simulink model "MPC_gamecontroller_LiDAR"  (Simulink 7.6)
settings: Solver=ode3  StartTime=0.0  StopTime=inf  FixedStep=.05  RelTol=1e-3
InitFcn:
  | a2g = 1/9.81;
  | r2d = 180/pi;
  | K_sr = 15.97;
  | neutral_steer = 103;
  | s2t = (pi/180)*(1/K_sr);
  | A_kt =[         0         0         0         0         0         0
  |          0   -3.5058   -1.6990  -25.6114   -2.2435         0
  |          0    2.2782   -4.2575  -64.1772   -5.6218         0
  |          0         0    1.0000         0         0         0
  |          0   -0.0158    0.0295    0.4442   -4.1900         0
  |          0         0         0         0    1.0000         0];
  | 
  | 
  | B_kt =[0
  |    23.7845
  |   -16.0342
  |          0
  |    17.5770
  |          0];
  | 
  | dt = 0.05;
  | measnoise_posX = 3.36;
  | measnoise_posY = 3.95;
  | measnoise_theta = 0.136;
  | measnoise_phi =  0.078;
  | measnoise_velocity = measnoise_posX*dt;
  | 
  | accelnoiseX = 0.97;
  | accelnoiseY = 1.36;
  | gyronoisetheta = 0.04;
  | gyronoisephi = 0.021;
  | 
  | anx = accelnoiseX^2;
  | any = accelnoiseY^2;
  | anxy = accelnoiseX*accelnoiseY;
  | gntheta = gyronoisetheta^2;
  | agthetax = gyronoisetheta*accelnoiseX;
  | agthetay = gyronoisetheta*accelnoiseY;
  | gnphi = gyronoisephi^2;
  | agphix = gyronoisephi*accelnoiseX;
  | agphiy = gyronoisephi*accelnoiseY;
  | gnthetaphi = gyronoisetheta*gyronoisephi;
  | 
  | A = [1 dt 0 0 0 0;...
  |         0 1 0 0 0 0;...
  |         0 0 1 dt 0 0;...
  |         0 0 0 1 0 0;...
  |         0 0 0 0 1 0;...
  |         0 0 0 0 0 1];
  | 
  | Sw = [anx*dt^4/4, anx*dt^3/2, anxy*dt^4/4, anxy*dt^3/2,  agthetax*dt^3/2, agphix*dt^3/2;...
  |       anx*dt^3/2, anx*dt^2,   anxy*dt^3/2, anxy*dt^2, agthetax*dt^2,   agphix*dt^2;...
  |       anxy*dt^4/4, anxy*dt^3/2, any*dt^4/4, any*dt^3/2,  agthetay*dt^3/2, agphiy*dt^3/2;...
  |       anxy*dt^3/2, anxy*dt^2,   any*dt^3/2, any*dt^2, agthetay*dt^2, agphiy*dt^2;...
  |       agthetax*dt^3/2, agthetax*dt^2, agthetay*dt^3/2, agthetay*dt^2, gntheta*dt^2, gnthetaphi*dt^2;...
  |       agphix*dt^3/2, agphix*dt^2, agphiy*dt^3/2, agphiy*dt^2, gnthetaphi*dt^2, gnphi*dt^2];
  | 
  | Sz =  [measnoise_posX^2, 0, 0, 0, 0, 0;...
  |          0, measnoise_velocity^2, 0, 0, 0, 0;...
  |          0, 0, measnoise_posY^2, 0, 0, 0;...
  |          0, 0, 0, measnoise_velocity^2, 0, 0;...
  |          0, 0, 0, 0, measnoise_theta^2, 0;...
  |          0, 0, 0, 0, 0, measnoise_phi^2];
  | 
  | load MPC_test_2
StartFcn:
  | Threshold = 12;
  | MaxCluster = 75;
  | Num_Beams = 726;
  | Road_Width = 10.25;
  | Cone_Area = 0.125;
  | Cone_Spacing = 4.42;
  | Scaling = 1.1;
  | areaBuffer = 0.125;
  | spacingBuffer = 0.035;
  | RoadfromConeoffset = 0.3;
  | threatThreshold = 1;
  | distThreshold = 10;
  | minSpeed = 2.0;
  | minDistance = 1.0;
  | threatConeAngle = 75;
  | allowableDistToCone = .01;
  | thresholdManueverAngle = 80;
  | maxStepSize = 1.0;
  | aspectRatioBuffer = 1;
  | javaaddpath({'/'});
  | import ClusterMethodWithFinal.*;
  | %import ClusterMethodWithNoFlicker.*;
  | %DataCluster = ClusterMethodWithNoFlicker(Threshold,MaxCluster,Scaling,...
  | %Road_Width,Cone_Area,Cone_Spacing,areaBuffer,spacingBuffer,RoadfromConeoffset,threatThreshold,...
  | %distThreshold,minSpeed,minDistance,threatConeAngle,allowableDistToCone,maxStepSize);
  | DataCluster = ClusterMethodWithFinal(Threshold,MaxCluster,Scaling,...
  | Road_Width,Cone_Area,Cone_Spacing,areaBuffer,spacingBuffer,RoadfromConeoffset,...
  | threatThreshold,distThreshold,minSpeed,minDistance,threatConeAngle,allowableDistToCone,...
  | thresholdManueverAngle,maxStepSize);
  | eml.extrinsic('evalin');
  | 
  | gd_scan(0);
StopFcn:
  | clear DataCluster;
  | clear Threshold;
  | clear MaxCluster;
  | clear Num_Beams;
  | clear Road_Width;
  | clear Cone_Area;
  | clear Cone_Spacing;
  | clear Scaling;
  | clear areaBuffer;
  | clear spacingBuffer;
  | clear RoadfromConeoffset;
  | clear threatThreshold;
  | clear distThreshold;
  | clear minSpeed;
  | clear minDistance;
  | clear threatConeAngle;
  | clear allowableDistToCone;
  | clear thresholdManueverAngle;
  | clear maxStepSize;
  | clear aspectRatioBuffer;
  | 
  | gd_scan(2);
undefined symbols (not defined in the file or in its folder): CR, serial
libraries: instrumentlib x3, realtime_pacer_lib x1, vrlib x1
settings Model: Creator=TCA  LastModifiedBy=ipainter  BufferReuse=off
settings OptimizationCC: BlockReduction=off  InlineParams=on  BufferReuse=off  InitFltsAndDblsToZero=on
settings DebuggingCC: AlgebraicLoopMsg=none  SolverPrmCheckMsg=none  InheritedTsInSrcMsg=none  UnconnectedInputMsg=none  UnconnectedOutputMsg=none  UnconnectedLineMsg=none  StrictBusMsg=Warning
settings SFSimCC: SimParseCustomCode=off

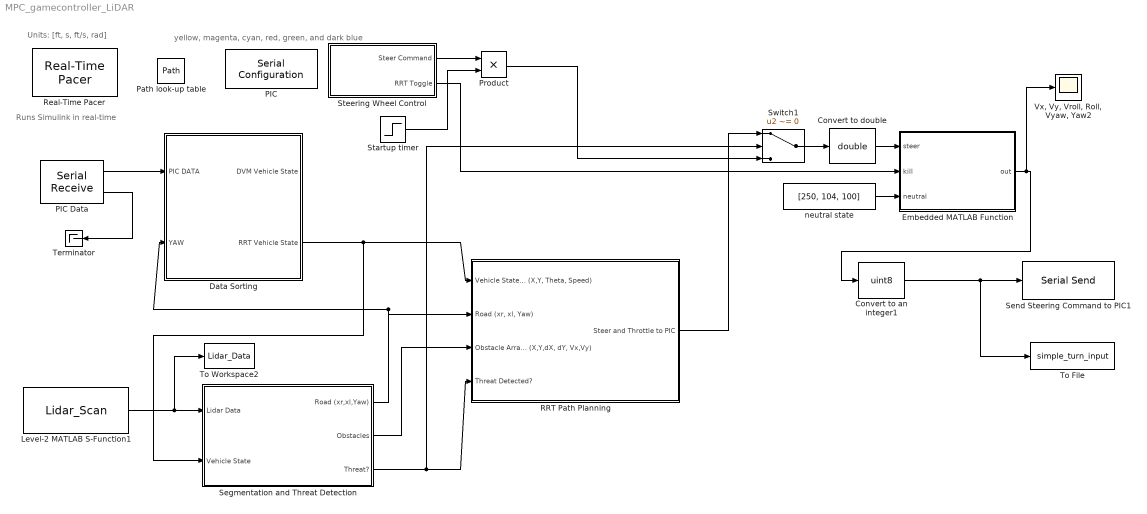
== system MPC_gamecontroller_LiDAR ==
  note: Runs Simulink
      |  in real-time
  note: Units: [ft, s, ft/s, rad]
  note: yellow, magenta, cyan, red, green, and dark blue
  Convert to an integer1 : DataTypeConversion  OutDataTypeStr=uint8  SampleTime=.05  SaturateOnIntegerOverflow=on  RndMeth=Zero
  Convert to double : DataTypeConversion  OutDataTypeStr=double  SampleTime=0.05  SaturateOnIntegerOverflow=on  RndMeth=Zero
  Data Sorting : Subsystem
  Embedded MATLAB Function : Stateflow chart  TreatAsAtomicUnit=on
  Level-2 MATLAB S-Function1 : M-S-Function  FunctionName=Lidar_Scan
  PIC : instrumentlib/Serial Configuration  Priority=-200000  DialogController=instrumentcreatedialog  DialogControllerArgs=DataTag0  ComPortMenu=<Please select a port...>  ComPort=COM5  ObjConstructor=serial('COM5');  BaudRate=9600  DataBits=8  Parity=none  StopBits=1  FlowControl=none  Timeout=10  ByteOrder=LittleEndian
  PIC Data : instrumentlib/Serial Receive  DialogController=instrumentcreatedialog  DialogControllerArgs=DataTag1  ComPortMenu=<Please select a port...>  ComPort=COM5  ObjConstructor=serial('COM5');  Terminator=CR ('\r')  DataSize="[1  16]"  DataType=uint8  EnableBlockingMode=off  ActionDataUnavailable=Output last received value  CustomValue=0  SampleTime=.05
  Path look-up table : DataStoreMemory  DataStoreName=Path  ReadBeforeWriteMsg=warning  WriteAfterWriteMsg=warning  WriteAfterReadMsg=warning  InitialValue=zeros(50, 6)  VectorParams1D=off
  Product : Product  RndMeth=Zero
  RRT Path Planning : Subsystem
  Real-Time Pacer : realtime_pacer_lib/Real-Time Pacer  simTimePerRealTime=1
  Segmentation and Threat Detection : Subsystem
  Send Steering Command to PIC1 : instrumentlib/Serial Send  DialogController=instrumentcreatedialog  DialogControllerArgs=DataTag2  ComPortMenu=<Please select a port...>  ComPort=COM5  ObjConstructor=serial('COM5');  Header=250  Terminator=<none>  EnableBlockingMode=off
  Startup timer : Step  Time=3  SampleTime=0
  Steering Wheel Control : Subsystem
  Switch1 : Switch  Criteria=u2 ~= 0
  Terminator : Terminator
  To File : ToFile  Filename=simple_turn_input  MatrixName=ST_input  SaveFormat=Timeseries
  To Workspace2 : ToWorkspace  VariableName=Lidar_Data  SampleTime=-1  SaveFormat=Structure With Time
  "Vx, Vy, Vroll, Roll, Vyaw, Yaw2" : Scope
      settings: TimeRange=10  YMax=30
  neutral state : Constant  Value=[250, 104, 100]
  wires:
  Convert to an integer1/1 -> To File/1, Send Steering Command to PIC1/1
  PIC Data/2 -> Terminator/1
  PIC Data/1 -> Data Sorting/1(PIC DATA)
  Segmentation and Threat Detection/2(Obstacles) -> RRT Path Planning/3("Obstacle Array (X,Y,dX, dY, Vx,Vy)")
  Segmentation and Threat Detection/1(Road (xr,xl,Yaw)) -> Data Sorting/2(" YAW"), RRT Path Planning/2("Road (xr, xl, Yaw)")
  RRT Path Planning/1(Steer and Throttle to PIC) -> Switch1/1
  Data Sorting/2(RRT Vehicle State) -> RRT Path Planning/1("Vehicle State (X,Y, Theta, Speed)"), Segmentation and Threat Detection/2(Vehicle State)
  neutral state/1 -> Embedded MATLAB Function/3(neutral)
  Embedded MATLAB Function/1(out) -> Convert to an integer1/1, "Vx, Vy, Vroll, Roll, Vyaw, Yaw2"/1
  Switch1/1 -> Convert to double/1
  Segmentation and Threat Detection/3(Threat?) -> Switch1/2, RRT Path Planning/4(Threat Detected?)
  Steering Wheel Control/1(Steer Command) -> Product/1
  Product/1 -> Switch1/3
  Startup timer/1 -> Product/2
  Steering Wheel Control/2(RRT Toggle) -> Embedded MATLAB Function/2(kill)
  Convert to double/1 -> Embedded MATLAB Function/1(steer)
  Level-2 MATLAB S-Function1/1 -> Segmentation and Threat Detection/1(Lidar Data), To Workspace2/1

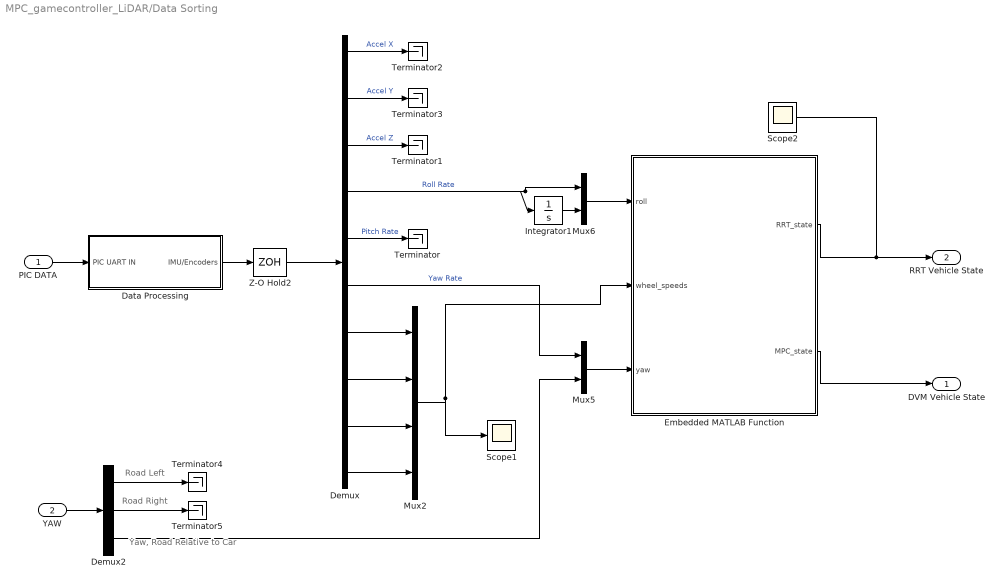
== system MPC_gamecontroller_LiDAR/Data Sorting ==
  note: Road Left
  note: Road Right
  note: Yaw, Road Relative to Car
  PIC DATA : Inport
  " YAW" : Inport  Port=2
  Data Processing : Subsystem
  Demux : Demux  Outputs=10
  Demux2 : Demux  Outputs=3
  Embedded MATLAB Function : Stateflow chart  TreatAsAtomicUnit=on
  Integrator1 : Integrator
  Mux2 : Mux
  Mux5 : Mux  Inputs=2
  Mux6 : Mux  Inputs=2
  Scope1 : Scope
      settings: SaveName=ScopeData3
  Scope2 : Scope
      settings: SaveName=ScopeData4
  Terminator{,1..5} (6 alike) : Terminator
  Z-O Hold2 : ZeroOrderHold  SampleTime=0.05
  DVM Vehicle State : Outport
  RRT Vehicle State : Outport  Port=2
  wires:
  Demux/6 -> Mux5/1  "Yaw Rate"
  Demux/2 -> Terminator3/1  "Accel Y"
  Demux/4 -> Mux6/1, Integrator1/1  "Roll Rate"
  Demux/5 -> Terminator/1  "Pitch Rate"
  Demux/7 -> Mux2/1
  Demux/8 -> Mux2/2
  Demux/9 -> Mux2/3
  Demux/10 -> Mux2/4
  Z-O Hold2/1 -> Demux/1
  Integrator1/1 -> Mux6/2
  Mux6/1 -> Embedded MATLAB Function/1(roll)
  Demux/1 -> Terminator2/1  "Accel X"
  Embedded MATLAB Function/2(MPC_state) -> DVM Vehicle State/1
  " YAW"/1 -> Demux2/1
  Demux/3 -> Terminator1/1  "Accel Z"
  Demux2/1 -> Terminator4/1
  Demux2/2 -> Terminator5/1
  Demux2/3 -> Mux5/2
  Mux5/1 -> Embedded MATLAB Function/3(yaw)
  Embedded MATLAB Function/1(RRT_state) -> RRT Vehicle State/1, Scope2/1
  Data Processing/1(IMU/Encoders) -> Z-O Hold2/1
  PIC DATA/1 -> Data Processing/1(PIC UART IN)
  Mux2/1 -> Embedded MATLAB Function/2(wheel_speeds), Scope1/1

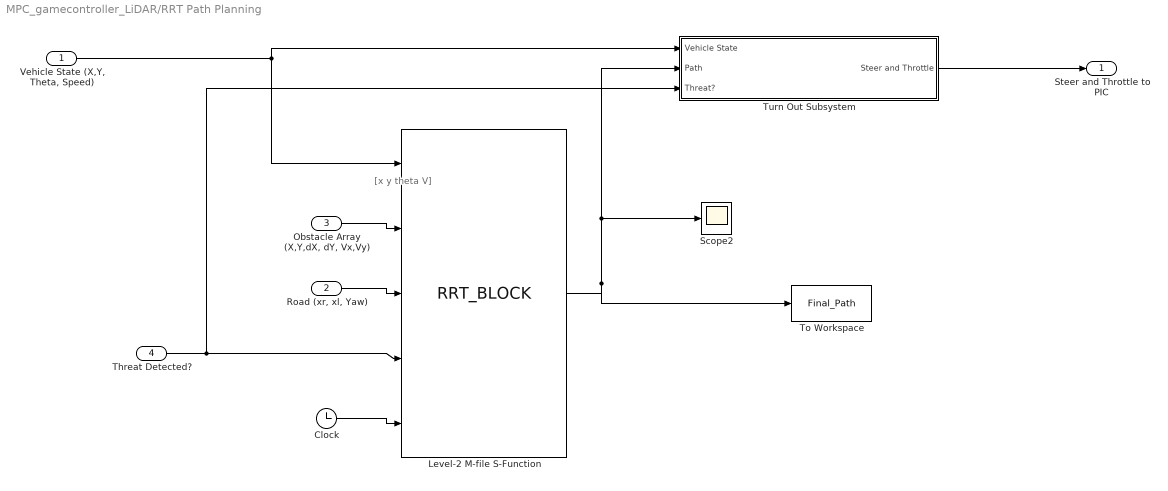
== system MPC_gamecontroller_LiDAR/RRT Path Planning ==
  note: [x y theta V]
  "Vehicle State (X,Y, Theta, Speed)" : Inport
  "Road (xr, xl, Yaw)" : Inport  Port=2
  "Obstacle Array (X,Y,dX, dY, Vx,Vy)" : Inport  Port=3
  Threat Detected? : Inport  Port=4
  Clock : Clock
      settings: Decimation=10
  Level-2 M-file S-Function : M-S-Function  FunctionName=RRT_BLOCK  Parameters=6
  Scope2 : Scope
      settings: SaveName=ScopeData5
  To Workspace : ToWorkspace  VariableName=Final_Path  SampleTime=-1  SaveFormat=Structure With Time
  Turn Out Subsystem : Subsystem
  Steer and Throttle to PIC : Outport
  wires:
  Clock/1 -> Level-2 M-file S-Function/5
  "Vehicle State (X,Y, Theta, Speed)"/1 -> Level-2 M-file S-Function/1, Turn Out Subsystem/1(Vehicle State)
  "Obstacle Array (X,Y,dX, dY, Vx,Vy)"/1 -> Level-2 M-file S-Function/2
  Turn Out Subsystem/1(Steer and Throttle) -> Steer and Throttle to PIC/1
  Threat Detected?/1 -> Level-2 M-file S-Function/4, Turn Out Subsystem/3(Threat?)
  "Road (xr, xl, Yaw)"/1 -> Level-2 M-file S-Function/3
  Level-2 M-file S-Function/1 -> Turn Out Subsystem/2(Path), Scope2/1, To Workspace/1

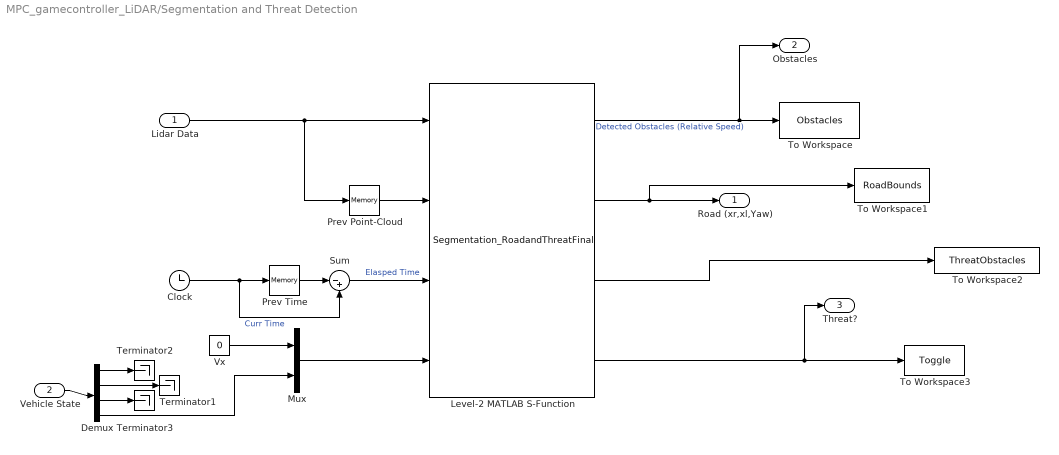
== system MPC_gamecontroller_LiDAR/Segmentation and Threat Detection ==
  Lidar Data : Inport
  Vehicle State : Inport  Port=2
  Clock : Clock
      settings: Decimation=10
  Demux : Demux
  Level-2 MATLAB S-Function : M-S-Function  FunctionName=Segmentation_RoadandThreatFinal
  Mux : Mux  Inputs=2
  Prev Point-Cloud : Memory
  Prev Time : Memory
  Sum : Sum  Inputs=|-+
  Terminator1 : Terminator
  Terminator2 : Terminator
  Terminator3 : Terminator
  To Workspace : ToWorkspace  VariableName=Obstacles  SampleTime=-1  SaveFormat=Structure With Time
  To Workspace1 : ToWorkspace  VariableName=RoadBounds  SampleTime=-1  SaveFormat=Structure With Time
  To Workspace2 : ToWorkspace  VariableName=ThreatObstacles  SampleTime=-1  SaveFormat=Structure With Time
  To Workspace3 : ToWorkspace  VariableName=Toggle  SampleTime=-1  SaveFormat=Structure With Time
  Vx : Constant  Value=0
  Road (xr,xl,Yaw) : Outport
  Obstacles : Outport  Port=2
  Threat? : Outport  Port=3
  wires:
  Prev Time/1 -> Sum/1
  Sum/1 -> Level-2 MATLAB S-Function/3  "Elasped Time"
  Clock/1 -> Prev Time/1, Sum/2  "Curr Time"
  Prev Point-Cloud/1 -> Level-2 MATLAB S-Function/2
  Level-2 MATLAB S-Function/1 -> To Workspace/1, Obstacles/1  "Detected Obstacles (Relative Speed)"
  Lidar Data/1 -> Prev Point-Cloud/1, Level-2 MATLAB S-Function/1
  Mux/1 -> Level-2 MATLAB S-Function/4
  Level-2 MATLAB S-Function/4 -> To Workspace3/1, Threat?/1
  Vx/1 -> Mux/1
  Vehicle State/1 -> Demux/1
  Demux/4 -> Mux/2
  Demux/1 -> Terminator2/1
  Demux/2 -> Terminator1/1
  Demux/3 -> Terminator3/1
  Level-2 MATLAB S-Function/2 -> Road (xr,xl,Yaw)/1, To Workspace1/1
  Level-2 MATLAB S-Function/3 -> To Workspace2/1

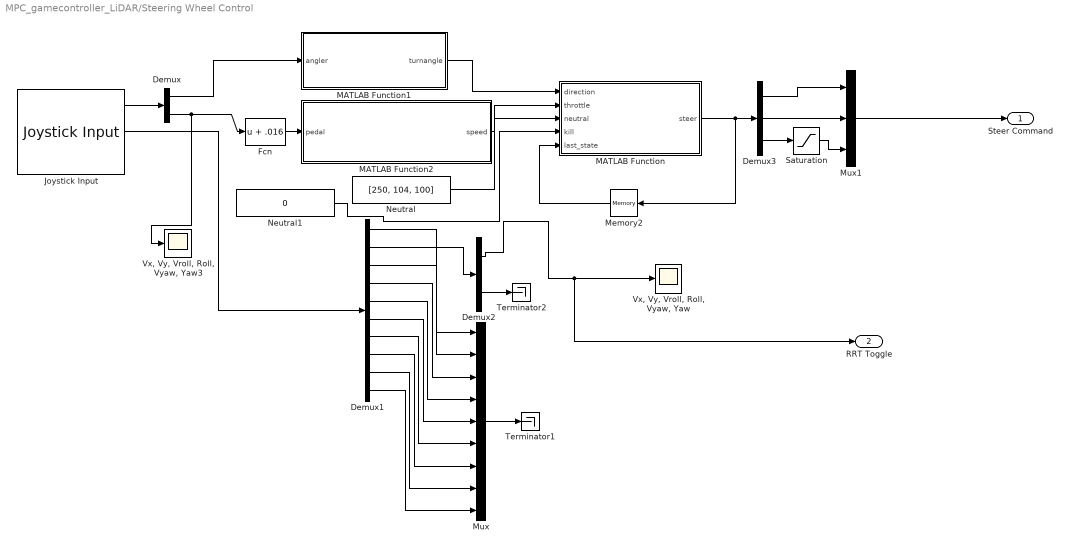
== system MPC_gamecontroller_LiDAR/Steering Wheel Control ==
  Demux : Demux  Outputs=2
  Demux1 : Demux  Outputs=10
  Demux2 : Demux  Outputs=2
  Demux3 : Demux  Outputs=3
  Fcn : Fcn  Expr=u + .016
  Joystick Input : vrlib/Joystick Input  joyid=1  adjustports=on  forcefeed=off
  MATLAB Function : Stateflow chart  TreatAsAtomicUnit=on
  MATLAB Function1 : Stateflow chart  TreatAsAtomicUnit=on
  MATLAB Function2 : Stateflow chart  TreatAsAtomicUnit=on
  Memory2 : Memory  X0=[250,104,100]  InheritSampleTime=on
  Mux : Mux  Inputs=9
  Mux1 : Mux  Inputs=3
  Neutral : Constant  Value=[250, 104, 100]
  Neutral1 : Constant  Value=0
  Saturation : Saturate  UpperLimit=200  LowerLimit=100
  Terminator1 : Terminator
  Terminator2 : Terminator
  "Vx, Vy, Vroll, Roll, Vyaw, Yaw" : Scope
      settings: TimeRange=10  YMax=30  SaveName=ScopeData7
  "Vx, Vy, Vroll, Roll, Vyaw, Yaw3" : Scope
      settings: TimeRange=10  YMax=30  SaveName=ScopeData6
  Steer Command : Outport
  RRT Toggle : Outport  Port=2
  wires:
  Joystick Input/1 -> Demux/1
  MATLAB Function2/1(speed) -> MATLAB Function/2(throttle)
  Neutral/1 -> MATLAB Function/3(neutral)
  Demux1/2 -> Demux2/1
  Demux2/1 -> "Vx, Vy, Vroll, Roll, Vyaw, Yaw"/1, RRT Toggle/1
  Demux2/2 -> Terminator2/1
  Demux1/1 -> Mux/1
  Demux1/3 -> Mux/2
  Demux1/4 -> Mux/3
  Demux1/5 -> Mux/4
  Demux1/6 -> Mux/5
  Demux1/7 -> Mux/6
  Demux1/8 -> Mux/7
  Demux1/9 -> Mux/8
  Demux1/10 -> Mux/9
  Mux/1 -> Terminator1/1
  Demux/2 -> "Vx, Vy, Vroll, Roll, Vyaw, Yaw3"/1, Fcn/1
  MATLAB Function1/1(turnangle) -> MATLAB Function/1(direction)
  Demux/1 -> MATLAB Function1/1(angler)
  Joystick Input/2 -> Demux1/1
  MATLAB Function/1(steer) -> Memory2/1, Demux3/1
  Memory2/1 -> MATLAB Function/5(last_state)
  Demux3/3 -> Saturation/1
  Saturation/1 -> Mux1/3
  Demux3/1 -> Mux1/1
  Mux1/1 -> Steer Command/1
  Neutral1/1 -> MATLAB Function/4(kill)
  Demux3/2 -> Mux1/2
  Fcn/1 -> MATLAB Function2/1(pedal)

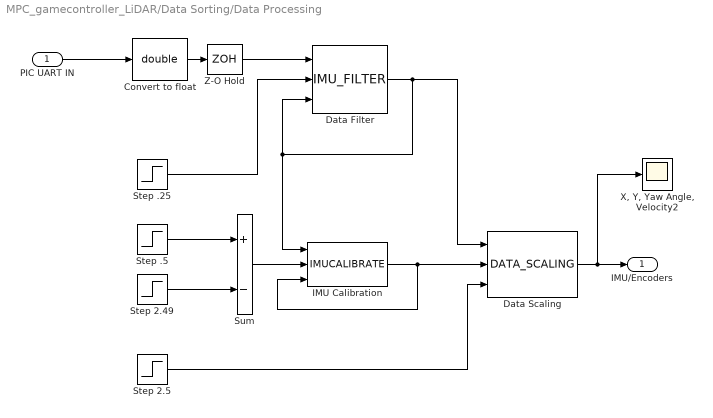
== system MPC_gamecontroller_LiDAR/Data Sorting/Data Processing ==
  PIC UART IN : Inport
  Convert to float : DataTypeConversion  OutDataTypeStr=double  SaturateOnIntegerOverflow=on  RndMeth=Zero
  Data Filter : M-S-Function  FunctionName=IMU_FILTER  Parameters=3
  "Data Scaling " : M-S-Function  FunctionName=DATA_SCALING  Parameters=3
  IMU Calibration : M-S-Function  FunctionName=IMUCALIBRATE  Parameters=3
  Step .25 : Step  Time=.25  SampleTime=0
  Step .5 : Step  Time=.5  SampleTime=0
  Step 2.49 : Step  Time=2.49  SampleTime=0
  Step 2.5 : Step  Time=2.5  SampleTime=0
  Sum : Sum  Inputs=+-
  "X, Y, Yaw Angle, Velocity2" : Scope
      settings: TimeRange=10  YMin=-1  YMax=1  SaveName=ScopeData9
  Z-O Hold : ZeroOrderHold  SampleTime=0.05
  IMU/Encoders : Outport
  wires:
  Convert to float/1 -> Z-O Hold/1
  Data Filter/1 -> "Data Scaling "/1, IMU Calibration/1, Data Filter/3
  IMU Calibration/1 -> IMU Calibration/3, "Data Scaling "/2
  Step .5/1 -> Sum/1
  Step 2.49/1 -> Sum/2
  Z-O Hold/1 -> Data Filter/1
  Step .25/1 -> Data Filter/2
  Sum/1 -> IMU Calibration/2
  Step 2.5/1 -> "Data Scaling "/3
  "Data Scaling "/1 -> IMU/Encoders/1, "X, Y, Yaw Angle, Velocity2"/1
  PIC UART IN/1 -> Convert to float/1

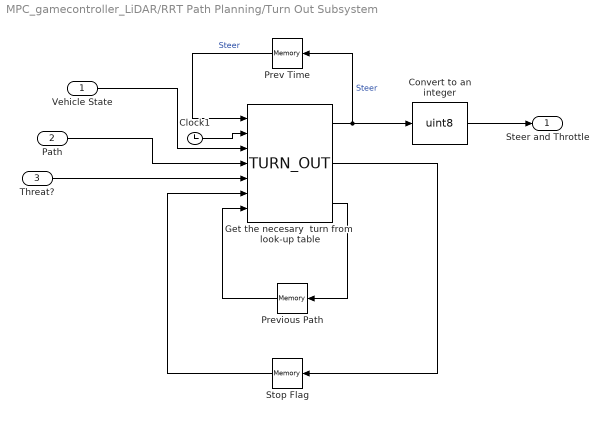
== system MPC_gamecontroller_LiDAR/RRT Path Planning/Turn Out Subsystem ==
  Vehicle State : Inport
  Path : Inport  Port=2
  Threat? : Inport  Port=3
  Clock1 : Clock
      settings: Decimation=10
  Convert to an integer : DataTypeConversion  OutDataTypeStr=uint8  SampleTime=.05  SaturateOnIntegerOverflow=on  RndMeth=Zero
  Get the necesary  turn from  look-up table : M-S-Function  FunctionName=TURN_OUT  Parameters=4
  Prev Time : Memory  X0=[250 0 0]
  Previous Path : Memory  X0=zeros(50,5)
  Stop Flag : Memory
  Steer and Throttle : Outport
  wires:
  Get the necesary  turn from  look-up table/1 -> Prev Time/1, Convert to an integer/1  "Steer"
  Convert to an integer/1 -> Steer and Throttle/1
  Prev Time/1 -> Get the necesary  turn from  look-up table/1  "Steer"
  Get the necesary  turn from  look-up table/2 -> Stop Flag/1
  Clock1/1 -> Get the necesary  turn from  look-up table/2
  Stop Flag/1 -> Get the necesary  turn from  look-up table/6
  Vehicle State/1 -> Get the necesary  turn from  look-up table/3
  Get the necesary  turn from  look-up table/3 -> Previous Path/1
  Previous Path/1 -> Get the necesary  turn from  look-up table/7
  Path/1 -> Get the necesary  turn from  look-up table/4
  Threat?/1 -> Get the necesary  turn from  look-up table/5

== matlab function Steering Wheel Control/MATLAB Function ==
  data: direction input double; steer output double; throttle input double; neutral input double; kill input double; last_state input double
function steer = controller_to_steer(direction,throttle,neutral,kill,last_state)
%#codegen
if(kill)
   steer = neutral;
else 
 steer = last_state;
 steer(2) = direction;
 steer(3) = throttle;   
end

== matlab function Data Sorting/Embedded MATLAB Function ==
  data: roll input double; wheel_speeds input double; yaw input double; RRT_state output double; MPC_state output double
% Updated: May 5th, 2013

% This function takes the scaled data from the IMU and uses it to determine
% the vehicle states for the RRT and the MPC.  Note that the state of the
% vehicle is always [0 0 Yaw V]  as the coordinate system is bases on the
% postion of the vehicle.

%DATA SORTING
function [RRT_state,MPC_state]  = data_sorting(roll,wheel_speeds,yaw)

%Calculate the vehicle velocity from the wheel encoder data.  this should
%be replaced with a more robust method as this neglects the fact that the
%vechicle may be turning as well as wheel slip
Index = find(wheel_speeds>17);
for n = 1:length(Index)
    wheel_speeds(Index(n)) = 15;
end

velocity = (wheel_speeds(1) + wheel_speeds(2) + wheel_speeds(3) + wheel_speeds(4))/4;


Phi_d = roll(1);            % Roll Rate
Phi = roll(2);              % Roll Angle  
Psi_d = yaw(1);             % Yaw Rate
Psi = yaw(2);               % Yaw angle of the road relative to the 
                            % centerline of the car
                            
Vy = velocity;              % Velocity of the vehicle

Vx = 0;                     % Always 0 as the Coordinates are 
                            % determined by the direction of the car


MPC_state = [Vy*(1/3.28), Vx*(1/3.28), Phi_d, Phi, Psi_d, Psi]';
RRT_state = [0, 0, Psi, velocity]';

== matlab function Steering Wheel Control/MATLAB Function1 ==
  data: angler input double; turnangle output double
function turnangle = scale_steer(angler)
%#codegen
if(angler>0)
    turnangle = 100+angler*(255-100);
elseif(angler<0)
    turnangle = 100+angler*100;
else 
    turnangle = 100;
end

== matlab function Steering Wheel Control/MATLAB Function2 ==
  data: pedal input double; speed output double
function speed = scale_throttle(pedal)
%#codegen
if(pedal>0)
    speed = 100-pedal*100;
elseif(pedal<0)
     speed = 100-pedal*(255-100);
else 
    speed = 100;
end

== matlab function Embedded MATLAB Function ==
  data: steer input double; kill input double; out output double; neutral input double
function out = fcn(steer,kill,neutral)
%#eml

if(kill)
    out = neutral;
else
    out = steer;
end

%end
